simulink model "schema_pendolo_PI"  (R2024b)
settings: Solver=VariableStepAuto  StartTime=0.0  StopTime=50.0  RelTol=1e-3
values from neighbouring files (symbols this model uses):
  A = sqrt(k1/k2)    [analisi_MMS.m]    (also in regolatore_Pendolo.m = [0 1 0 0 ;       0 0 -m*g/M 0;       0 0 0 1 ;       0 0 (M+; run_ARE.m = [1 1 0; 0 1 1; 1 0 1])
  B = k1/sqrt(2*k2*m)    [analisi_MMS.m]    (also in regolatore_Pendolo.m = [ 0      0 ;       1/M -m*l/M*j_p; run_ARE.m = [1 1 0;3 1 0; 0 0 1])
  C_tilde = -C    [regolatore_Pendolo.m]
  F = [A-G0*C+B*K P-G0*Q_tilde+B*(G-K*T) ; -G1*C S-G1*Q_tilde]    [regolatore_Pendolo.m]    (also in regolatore_robot.m = [F1*qp_1 ; F2*qp_2])
  G0 = G_e(1:4,:)    [regolatore_Pendolo.m]
  G1 = G_e(5:7,:)    [regolatore_Pendolo.m]
  H = [K G-K*T]    [regolatore_Pendolo.m]
settings Model: Creator=david  LastModifiedBy=david

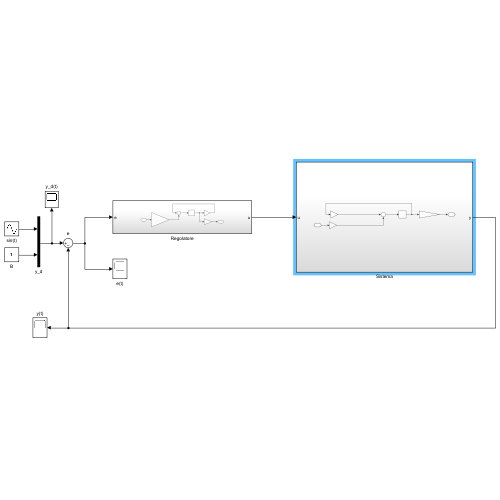
[thumbnail: Simulink's stored preview of the top-level diagram]
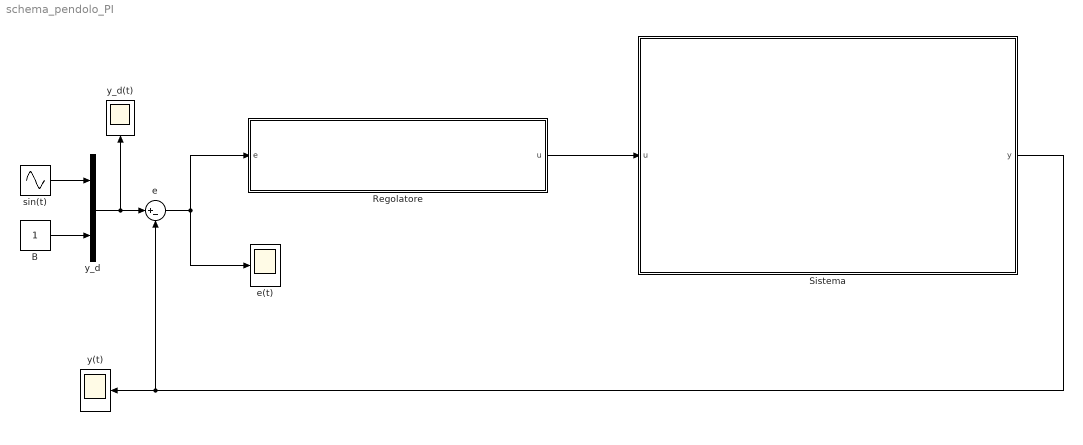
== system schema_pendolo_PI ==
  B : Constant
  Regolatore : Subsystem
  Sistema : Subsystem
  e : Sum  Inputs=|+-
  e(t) : Scope
  sin(t) : Sin  SampleTime=0
  y(t) : Scope
  y_d : Mux  Inputs=2
  y_d(t) : Scope
  wires:
  sin(t)/1 -> y_d/1
  B/1 -> y_d/2
  y_d/1 -> e/1, y_d(t)/1
  e/1 -> Regolatore/1(e), e(t)/1
  Regolatore/1(u) -> Sistema/1(u)
  Sistema/1(y) -> e/2, y(t)/1

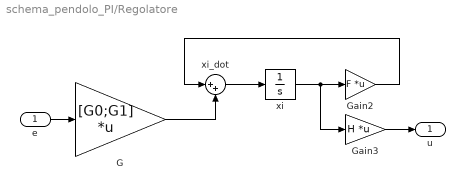
== system schema_pendolo_PI/Regolatore ==
  e : Inport
  G : Gain  Gain=[G0;G1]  Multiplication=Matrix(K*u)
  Gain2 : Gain  Gain=F  Multiplication=Matrix(K*u)
  Gain3 : Gain  Gain=H  Multiplication=Matrix(K*u)
  xi : Integrator
  xi_dot : Sum  Inputs=|++
  u : Outport
  wires:
  e/1 -> G/1
  G/1 -> xi_dot/2
  xi_dot/1 -> xi/1
  xi/1 -> Gain2/1, Gain3/1
  Gain2/1 -> xi_dot/1
  Gain3/1 -> u/1

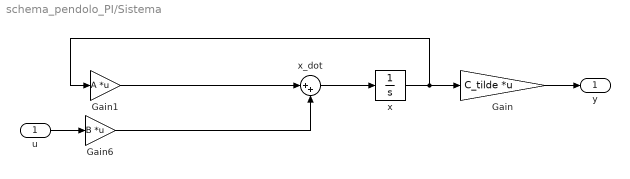
== system schema_pendolo_PI/Sistema ==
  u : Inport
  Gain : Gain  Gain=C_tilde  Multiplication=Matrix(K*u)
  Gain1 : Gain  Gain=A  Multiplication=Matrix(K*u)
  Gain6 : Gain  Gain=B  Multiplication=Matrix(K*u)
  x : Integrator
  x_dot : Sum  Inputs=|++
  y : Outport
  wires:
  u/1 -> Gain6/1
  Gain1/1 -> x_dot/1
  x_dot/1 -> x/1
  x/1 -> Gain/1, Gain1/1
  Gain/1 -> y/1
  Gain6/1 -> x_dot/2
